simulink subsystem "EIS"  (R2022a)
settings: Solver=VariableStepAuto  StartTime=0.0  StopTime=10.0  RelTol=1e-3
libraries: fl_lib x5, nesl_utility x4, ee_lib x1
settings Model: Creator=mateu  LastModifiedBy=mateu

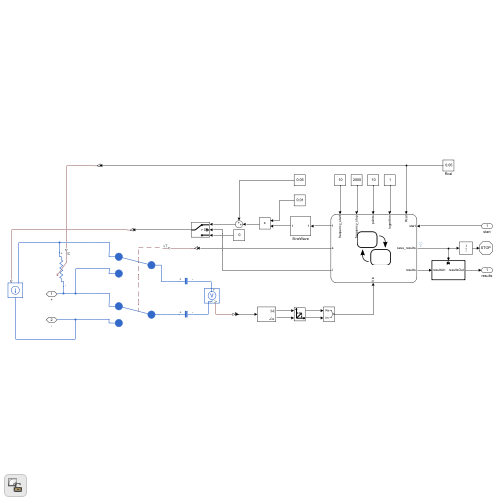
[thumbnail: Simulink's stored preview of the top-level diagram]
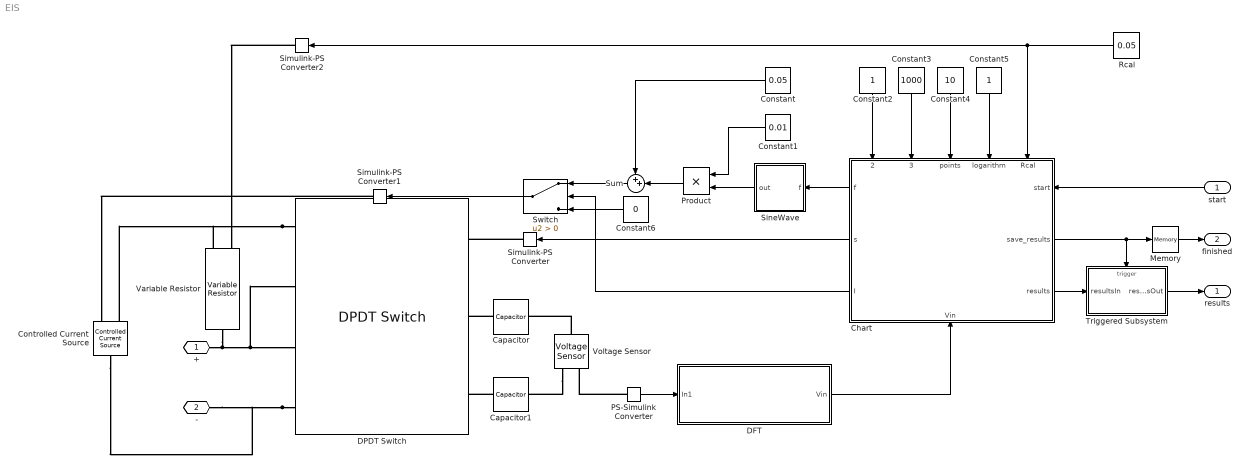
== system EIS ==
  start : Inport
  Capacitor : fl_lib/Electrical/Electrical Elements/Capacitor  c=2.2 uF  r=1e-6 Ohm  g=0 1/Ohm  i_specify=off  i_priority=None  i=0 A  i_nominal_specify=off  i_nominal_unit=A  i_nominal_value=1  v_specify=off  v_priority=None  v=0 V  v_nominal_specify=off  v_nominal_unit=V  v_nominal_value=1  vc_specify=off  vc_priority=High  vc=0 V  vc_nominal_specify=off  vc_nominal_unit=V  vc_nominal_value=1
      settings: SourceProductBaseCode=PW,SS,VE
  Capacitor1 : fl_lib/Electrical/Electrical Elements/Capacitor  c=2.2 uF  r=1e-6 Ohm  g=0 1/Ohm  i_specify=off  i_priority=None  i=0 A  i_nominal_specify=off  i_nominal_unit=A  i_nominal_value=1  v_specify=off  v_priority=None  v=0 V  v_nominal_specify=off  v_nominal_unit=V  v_nominal_value=1  vc_specify=off  vc_priority=High  vc=0 V  vc_nominal_specify=off  vc_nominal_unit=V  vc_nominal_value=1
      settings: SourceProductBaseCode=PW,SS,VE
  Chart : Stateflow chart  TreatAsAtomicUnit=on
      settings: PortSchema="{\"entries\":[{\"content\":{\"sides\":[{\"content\":{\"connectorIds\":[\"In6\",\"Out4\",\"Out5\"]},\"type\":\"ConnectorPlacement.EquallySpacedRectSide\",\"uuid\":\"c3a298c3-ea46-4ce2-abab-210af68c3657\"},{\"content\":{\"connectorIds\":[\"Out1\",\"Out2\",\"Out3\"],\"side\":\"RIGHT\"},\"type\":\"ConnectorPlacement.EquallySpacedRectSide\",\"uuid\":\"0861f50c-9fd4-48fa-8641-6baea44f4b8e\"},{\"content\":{\"connectorIds\":[\"In7\",\"In4\",\"In5\",\"In3\",\"In2\"],\"side\":\"TOP\"},\"type\":\"ConnectorPlacement.EquallySpacedRectSide\",\"uuid\":\"517d3c9b-6db8-41ea-a262-813b7ee62be9\"},{\"content\":{\"connectorIds\":[\"In1\"],\"side\":\"BOTTOM\"},\"type\":\"ConnectorPlacement.EquallySpacedRectSide\",\"uuid\":\"f85d206b-1290-4ef7-9258-619bcd5ec841\"}]},\"type\":\"ConnectorPlacement.EquallySpacedConnector\",\"uuid\":\"1da80215-03d8-4829-87ae-f0c66c5ff921\"}],\"packageUris\":[\"http://schema.mathworks.com/mf0/Connector/R2020b\"],\"version\":\"1.0\"}"
  Constant : Constant  Value=0.05
  Constant1 : Constant  Value=0.01
  Constant2 : Constant
  Constant3 : Constant  Value=1000
  Constant4 : Constant  Value=10
  Constant5 : Constant
  Constant6 : Constant  Value=0
  Controlled Current Source : fl_lib/Electrical/Electrical Sources/Controlled Current Source
      settings: SourceProductBaseCode=PW,SS,VE
  DFT : Subsystem
  DPDT Switch : ee_lib/Switches & Breakers/DPDT Switch  R_closed=0.01 Ohm  G_open=1e-6 S  Threshold=0.5 V  Width=0 V  model_dynamics=0  t_on=1e-3 s  t_off=1e-3 s  initial_vT=0 V
      settings: SourceProductBaseCode=PS  InternalSimscapePortConfiguration="{\"Bottom\":[],\"Left\":[{\"id\":\"vT\",\"label\":\"vT\",\"type\":\"input\"},{\"id\":\"p1\",\"label\":\"\",\"type\":\"foundation.electrical.electrical\"},{\"id\":\"p2\",\"label\":\"\",\"type\":\"foundation.electrical.electrical\"}],\"Right\":[{\"id\":\"n11\",\"label\":\"\",\"type\":\"foundation.electrical.electrical\"},{\"id\":\"n12\",\"label\":\"\",\"type\":\"foundation.electrical.electrical\"},{\"id\":\"n21\",\"label\":\"\",\"type\":\"foundation.electrical.electrical\"},{\"id\":\"n22\",\"label\":\"\",\"type\":\"foundation.electrical.electrical\"}],\"Top\":[]}"
  Memory : Memory
  PS-Simulink Converter : nesl_utility/PS-Simulink Converter  PhysicalDomain=network_engine_domain  SubClassName=ps_output  LeftPortType=input  RightPortType=output  PseudoPeriodic=off  Frequencies=[]  VectorFormat=inherit  Unit=inherit  AffineConversion=off
      settings: SourceProductBaseCode=SS,PW,VE
  Product : Product
  Rcal : Constant  Value=0.05
  Simulink-PS Converter : nesl_utility/Simulink-PS Converter  PhysicalDomain=network_engine_domain  SubClassName=ps_input  LeftPortType=input  RightPortType=output  PseudoPeriodic=off  Frequencies=[]  NoiseDistribution=none  NoiseParameters=[]  Unit=1  AffineConversion=off  FilteringAndDerivatives=provide  SimscapeFilterOrder=1  InputFilterTimeConstant=0.001  UdotUserProvided=0
      settings: SourceProductBaseCode=SS,PW,VE
  Simulink-PS Converter1 : nesl_utility/Simulink-PS Converter  PhysicalDomain=network_engine_domain  SubClassName=ps_input  LeftPortType=input  RightPortType=output  PseudoPeriodic=off  Frequencies=[]  NoiseDistribution=none  NoiseParameters=[]  Unit=1  AffineConversion=off  FilteringAndDerivatives=provide  SimscapeFilterOrder=1  InputFilterTimeConstant=0.001  UdotUserProvided=0
      settings: SourceProductBaseCode=SS,PW,VE
  Simulink-PS Converter2 : nesl_utility/Simulink-PS Converter  PhysicalDomain=network_engine_domain  SubClassName=ps_input  LeftPortType=input  RightPortType=output  PseudoPeriodic=off  Frequencies=[]  NoiseDistribution=none  NoiseParameters=[]  Unit=1  AffineConversion=off  FilteringAndDerivatives=provide  SimscapeFilterOrder=1  InputFilterTimeConstant=0.001  UdotUserProvided=0
      settings: SourceProductBaseCode=SS,PW,VE
  SineWave : Subsystem
  Sum : Sum  Inputs=++|
  Switch : Switch  Criteria=u2 > Threshold  SaturateOnIntegerOverflow=off  InputSameDT=off
  Triggered Subsystem : Subsystem  TreatAsAtomicUnit=on
  Variable Resistor : fl_lib/Electrical/Electrical Elements/Variable Resistor  Rmin=0 Ohm  i_specify=off  i_priority=None  i=0 A  i_nominal_specify=off  i_nominal_unit=A  i_nominal_value=1  v_specify=off  v_priority=None  v=0 V  v_nominal_specify=off  v_nominal_unit=V  v_nominal_value=1
      settings: SourceProductBaseCode=PW,SS,VE
  Voltage Sensor : fl_lib/Electrical/Electrical Sensors/Voltage Sensor
      settings: SourceProductBaseCode=PW,SS,VE
  + : PMIOPort  Side=Left
  - : PMIOPort  Port=2  Side=Left
  results : Outport
  finished : Outport  Port=2
  wires:
  Constant6/1 -> Switch/3
  Constant5/1 -> Chart/4(logarithm)
  Chart/1(f) -> SineWave/1(f)
  Product/1 -> Sum/2
  Constant3/1 -> Chart/3(frequency_stop)
  Chart/2(s) -> Simulink-PS Converter/1
  Rcal/1 -> Chart/7(Rcal), Simulink-PS Converter2/1
  DFT/1(Vin) -> Chart/1(Vin)
  Constant/1 -> Sum/1
  Constant1/1 -> Product/1
  Constant2/1 -> Chart/2(frequency_start)
  Constant4/1 -> Chart/5(points)
  SineWave/1(out) -> Product/2
  Sum/1 -> Switch/1
  Switch/1 -> Simulink-PS Converter1/1
  Chart/3(I) -> Switch/2
  PS-Simulink Converter/1 -> DFT/1(In1)
  start/1 -> Chart/6(start)
  Triggered Subsystem/1(resultsOut) -> results/1
  Chart/5(results) -> Triggered Subsystem/1(resultsIn)
  Chart/4(save_results) -> Triggered Subsystem/Trigger, Memory/1
  Memory/1 -> finished/1
  connections:
  DPDT Switch/RConn4 -- Controlled Current Source/LConn1 -- -/RConn1
  +/RConn1 -- DPDT Switch/RConn2 -- DPDT Switch/RConn3 -- Variable Resistor/RConn1
  DPDT Switch/RConn1 -- Variable Resistor/LConn2 -- Controlled Current Source/RConn2
  Simulink-PS Converter2/RConn1 -- Variable Resistor/LConn1
  Voltage Sensor/RConn2 -- Capacitor1/RConn1
  Capacitor1/LConn1 -- DPDT Switch/LConn3
  Simulink-PS Converter1/RConn1 -- Controlled Current Source/RConn1
  Simulink-PS Converter/RConn1 -- DPDT Switch/LConn1
  Capacitor/LConn1 -- DPDT Switch/LConn2
  Voltage Sensor/LConn1 -- Capacitor/RConn1
  PS-Simulink Converter/LConn1 -- Voltage Sensor/RConn1

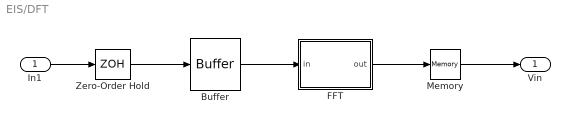
== system EIS/DFT ==
  In1 : Inport
  Buffer : Buffer  OutputFrames=off
  FFT : MATLAB Function  TreatAsAtomicUnit=on
  Memory : Memory
  Zero-Order Hold : ZeroOrderHold  SampleTime=1e-4
  Vin : Outport
  wires:
  Memory/1 -> Vin/1
  Zero-Order Hold/1 -> Buffer/1
  FFT/1(out) -> Memory/1
  Buffer/1 -> FFT/1(in)
  In1/1 -> Zero-Order Hold/1

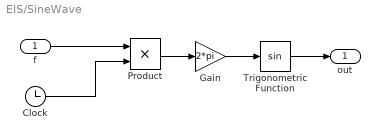
== system EIS/SineWave ==
  f : Inport
  Clock : Clock
  Gain : Gain  Gain=2*pi
  Product : Product
  Trigonometric Function : Trigonometry
  out : Outport
  wires:
  Gain/1 -> Trigonometric Function/1
  Product/1 -> Gain/1
  Clock/1 -> Product/2
  Trigonometric Function/1 -> out/1
  f/1 -> Product/1

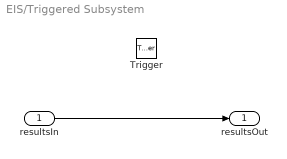
== system EIS/Triggered Subsystem ==
  resultsIn : Inport
  Trigger : TriggerPort  TriggerType=either  VariantControl=(inherit)  PortDimensions=1
  resultsOut : Outport
  wires:
  resultsIn/1 -> resultsOut/1

== matlab function EIS/DFT/FFT ==
  data: in input; out output
function out = fcn(in)

y = fft(in);                              % Compute DFT of x
m = abs(y);                               % Magnitude
y(m<1e-6) = 0;
p = unwrap(angle(y));                     % Phase

[mag,idx] = max(m);
out = mag*exp(1i*p(idx(1)));

== stateflow chart EIS/Chart ==
  settings: updateMethod=DISCRETE  sampleTime=0.001
  state Saving
  state Switching
  state Ready
    f=0; s=0; I=0;
  state StartSweep
  state SetFrequency
  state Measuring
  Switching -> Saving [order 2] : {
      | s=0;
      | Z(1:n) = V(1:n,2)./V(1:n,1)*Rcal;
      | results = [Z,transpose(f_list)];
      | save_results=1;
      | }
  Saving -> Ready : [after(1,msec)]
      | {
      | results=[];
      | save_results=0;
      | }
  Switching -> StartSweep [order 1] : [s==0]
      | {
      | s=1;
      | }
  (junction 32) -> Switching [order 1] : [i_f==n]{f=0;I=0;}
  (default) -> Ready
  SetFrequency -> Measuring : {
      | i_f=i_f+1;
      | f=f_list(i_f);
      | }
  Ready -> (junction 5) : [start==1]
      | {
      | n=points;
      | f_start=frequency_start;
      | f_stop=frequency_stop;
      | logen=logarithm;
      | V=complex(zeros(n,2));
      | Z=complex(zeros(n,1));
      | }
  (junction 5) -> StartSweep [order 1] : [logen~=1]
      | {
      | f_list = linspace(f_start,f_stop,n);
      | }
  Measuring -> (junction 32) : [after(10/f,sec)]
      | {
      | V(i_f,s+1)=Vin;
      | i_f=i_f+1;
      | }
  StartSweep -> SetFrequency : [after(1,sec)]
      | {
      | I=1;
      | i_f=0;
      | }
  (junction 5) -> StartSweep [order 2] : {
      | f_list=logspace(log10(f_start),log10(f_stop),n);
      | }
  (junction 32) -> SetFrequency [order 2]
  data: Vin input; frequency_start input; frequency_stop input; logarithm input; points input; start input; f_start local; f_stop local; i_f local; logen local; n local; Rcal input; V local size=[1000 2]; f output; s output; I output; save_results output; f_list local size=[1 1000]; Z local size=[1000 1]; results output size=[1000 2]
